simulink model "blob_analysis"  (Simulink 7.6)
settings: Solver=FixedStepDiscrete  StartTime=0.0  StopTime=0  FixedStep=1/30  RelTol=1e-3
values from neighbouring files (symbols this model uses):
  Iter_Segment_Thresh = 60    [VisionConstants.m]
undefined symbols (not defined in the file or in its folder): black_al, black_au, black_bl, black_bu, blue_al, blue_au, blue_bl, blue_bu, green_al, green_au, green_bl, green_bu, orange_al, orange_au, orange_bl, orange_bu, Rec, red_al, red_au, red_bl, red_bu, SDTV, white_al, white_au, white_bl, white_bu, yellow_al, yellow_au, yellow_bl, yellow_bu
libraries: vipgeotforms x21, vipconversions x14
(part 1 of 5)
settings Model: Creator=auvt  LastModifiedBy=auvt
settings RTWCC: TargetLang=C++

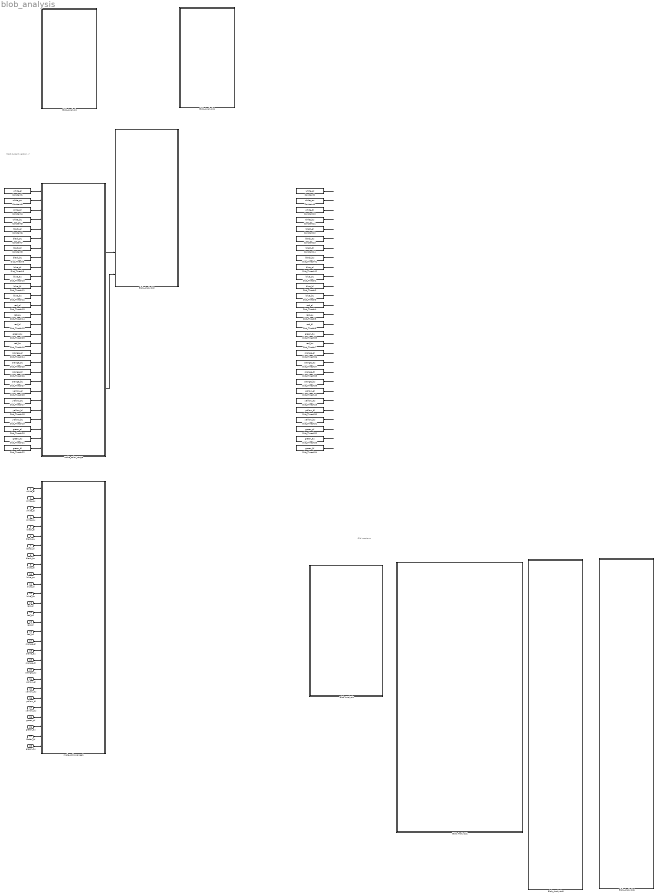
== system blob_analysis ==
  note: Old versions
  note: Most current version ->
  white_al : Inport
  white_au : Inport  Port=2
  white_bl : Inport  Port=3
  white_bu : Inport  Port=4
  black_al : Inport  Port=5
  black_au : Inport  Port=6
  black_bl : Inport  Port=7
  black_bu : Inport  Port=8
  blue_al : Inport  Port=9
  blue_au : Inport  Port=10
  blue_bl : Inport  Port=11
  blue_bu : Inport  Port=12
  red_al : Inport  Port=13
  red_au : Inport  Port=14
  red_bl : Inport  Port=15
  red_bu : Inport  Port=16
  orange_al : Inport  Port=17
  orane_au : Inport  Port=18
  orange_bl : Inport  Port=19
  orange_bu : Inport  Port=20
  yellow_al : Inport  Port=21
  yellow_au : Inport  Port=22
  yellow_bl : Inport  Port=23
  yellow_bu : Inport  Port=24
  green_al : Inport  Port=25
  green_au : Inport  Port=26
  breen_bl : Inport  Port=27
  green_bu : Inport  Port=28
  Blob Analysis : Subsystem
  Blob Analysis1 : Subsystem
  Blob_Analysis : Subsystem  TreatAsAtomicUnit=on
  Blob_Analysis1 : Subsystem  TreatAsAtomicUnit=on
  Blob_Analysis2 : Subsystem  TreatAsAtomicUnit=on
  Blob_Analysis5 : Subsystem  TreatAsAtomicUnit=on
  Blob_Analysis6 : Subsystem  TreatAsAtomicUnit=on
  Constant1 : Constant  Value=white_al  SampleTime=-1
  Constant10 : Constant  Value=white_bl  SampleTime=-1
  Constant11 : Constant  Value=white_bu  SampleTime=-1
  Constant12 : Constant  Value=black_al  SampleTime=-1
  Constant13 : Constant  Value=black_au  SampleTime=-1
  Constant14 : Constant  Value=black_bl  SampleTime=-1
  Constant2 : Constant  Value=white_al  SampleTime=-1
  Constant3 : Constant  Value=white_au  SampleTime=-1
  Constant4 : Constant  Value=white_bl  SampleTime=-1
  Constant5 : Constant  Value=white_bu  SampleTime=-1
  Constant6 : Constant  Value=black_al  SampleTime=-1
  Constant7 : Constant  Value=black_au  SampleTime=-1
  Constant8 : Constant  Value=black_bl  SampleTime=-1
  Constant9 : Constant  Value=white_au  SampleTime=-1
  Dist_Thresh1 : Constant  Value=blue_au  SampleTime=-1
  Dist_Thresh10 : Constant  Value=blue_au  SampleTime=-1
  Dist_Thresh11 : Constant  Value=blue_bl  SampleTime=-1
  Dist_Thresh12 : Constant  Value=blue_bu  SampleTime=-1
  Dist_Thresh13 : Constant  Value=red_al  SampleTime=-1
  Dist_Thresh14 : Constant  Value=red_au  SampleTime=-1
  Dist_Thresh15 : Constant  Value=red_bl  SampleTime=-1
  Dist_Thresh16 : Constant  Value=red_bu  SampleTime=-1
  Dist_Thresh17 : Constant  Value=yellow_au  SampleTime=-1
  Dist_Thresh18 : Constant  Value=yellow_bl  SampleTime=-1
  Dist_Thresh19 : Constant  Value=yellow_bu  SampleTime=-1
  Dist_Thresh2 : Constant  Value=blue_bl  SampleTime=-1
  Dist_Thresh20 : Constant  Value=green_al  SampleTime=-1
  Dist_Thresh21 : Constant  Value=green_au  SampleTime=-1
  Dist_Thresh22 : Constant  Value=green_bl  SampleTime=-1
  Dist_Thresh23 : Constant  Value=green_bu  SampleTime=-1
  Dist_Thresh24 : Constant  Value=orange_al  SampleTime=-1
  Dist_Thresh25 : Constant  Value=orange_au  SampleTime=-1
  Dist_Thresh26 : Constant  Value=orange_bl  SampleTime=-1
  Dist_Thresh27 : Constant  Value=orange_bu  SampleTime=-1
  Dist_Thresh28 : Constant  Value=yellow_al  SampleTime=-1
  Dist_Thresh29 : Constant  Value=yellow_au  SampleTime=-1
  Dist_Thresh3 : Constant  Value=blue_bu  SampleTime=-1
  Dist_Thresh30 : Constant  Value=yellow_bl  SampleTime=-1
  Dist_Thresh31 : Constant  Value=yellow_bu  SampleTime=-1
  Dist_Thresh32 : Constant  Value=green_al  SampleTime=-1
  Dist_Thresh33 : Constant  Value=green_au  SampleTime=-1
  Dist_Thresh34 : Constant  Value=green_bl  SampleTime=-1
  Dist_Thresh35 : Constant  Value=green_bu  SampleTime=-1
  Dist_Thresh36 : Constant  Value=orange_al  SampleTime=-1
  Dist_Thresh37 : Constant  Value=orange_au  SampleTime=-1
  Dist_Thresh38 : Constant  Value=orange_bl  SampleTime=-1
  Dist_Thresh39 : Constant  Value=orange_bu  SampleTime=-1
  Dist_Thresh4 : Constant  Value=red_al  SampleTime=-1
  Dist_Thresh40 : Constant  Value=yellow_al  SampleTime=-1
  Dist_Thresh41 : Constant  Value=black_bu  SampleTime=-1
  Dist_Thresh42 : Constant  Value=blue_al  SampleTime=-1
  Dist_Thresh5 : Constant  Value=red_au  SampleTime=-1
  Dist_Thresh6 : Constant  Value=red_bl  SampleTime=-1
  Dist_Thresh7 : Constant  Value=red_bu  SampleTime=-1
  Dist_Thresh8 : Constant  Value=black_bu  SampleTime=-1
  Dist_Thresh9 : Constant  Value=blue_al  SampleTime=-1
  make_color_range : Stateflow chart  TreatAsAtomicUnit=on
  make_color_range1 : Stateflow chart  TreatAsAtomicUnit=on
  wires:
  Constant1/1 -> make_color_range/1(white_al)
  Dist_Thresh22/1 -> make_color_range/28(green_bu)
  Constant3/1 -> make_color_range/2(white_au)
  Constant4/1 -> make_color_range/3(white_bl)
  Constant5/1 -> make_color_range/4(white_bu)
  Constant6/1 -> make_color_range/5(black_al)
  Constant7/1 -> make_color_range/6(black_au)
  Constant8/1 -> make_color_range/7(black_bl)
  Dist_Thresh8/1 -> make_color_range/8(black_bu)
  Dist_Thresh9/1 -> make_color_range/9(blue_al)
  Dist_Thresh10/1 -> make_color_range/10(blue_au)
  Dist_Thresh11/1 -> make_color_range/11(blue_bl)
  Dist_Thresh12/1 -> make_color_range/12(blue_bu)
  Dist_Thresh13/1 -> make_color_range/13(red_al)
  Dist_Thresh14/1 -> make_color_range/14(red_au)
  Dist_Thresh15/1 -> make_color_range/15(red_bl)
  Dist_Thresh23/1 -> make_color_range/16(red_bu)
  Dist_Thresh16/1 -> make_color_range/17(orange_al)
  Dist_Thresh24/1 -> make_color_range/18(orange_au)
  Dist_Thresh25/1 -> make_color_range/19(orange_bl)
  Dist_Thresh26/1 -> make_color_range/20(orange_bu)
  Dist_Thresh27/1 -> make_color_range/21(yellow_al)
  Dist_Thresh28/1 -> make_color_range/22(yellow_au)
  Dist_Thresh17/1 -> make_color_range/23(yellow_bl)
  Dist_Thresh18/1 -> make_color_range/24(yellow_bu)
  Dist_Thresh19/1 -> make_color_range/25(green_al)
  Dist_Thresh20/1 -> make_color_range/26(green_au)
  Dist_Thresh21/1 -> make_color_range/27(green_bl)
  Constant2/1 -> ?
  Dist_Thresh34/1 -> ?
  Constant9/1 -> ?
  Constant10/1 -> ?
  Constant11/1 -> ?
  Constant12/1 -> ?
  Constant13/1 -> ?
  Constant14/1 -> ?
  Dist_Thresh41/1 -> ?
  Dist_Thresh42/1 -> ?
  Dist_Thresh1/1 -> ?
  Dist_Thresh2/1 -> ?
  Dist_Thresh3/1 -> ?
  Dist_Thresh4/1 -> ?
  Dist_Thresh5/1 -> ?
  Dist_Thresh6/1 -> ?
  Dist_Thresh35/1 -> ?
  Dist_Thresh7/1 -> ?
  Dist_Thresh36/1 -> ?
  Dist_Thresh37/1 -> ?
  Dist_Thresh38/1 -> ?
  Dist_Thresh39/1 -> ?
  Dist_Thresh40/1 -> ?
  Dist_Thresh29/1 -> ?
  Dist_Thresh30/1 -> ?
  Dist_Thresh31/1 -> ?
  Dist_Thresh32/1 -> ?
  Dist_Thresh33/1 -> ?
  make_color_range/1(a_range) -> Blob_Analysis2/6(a_range)
  make_color_range/2(b_range) -> Blob_Analysis2/7(b_range)
  white_al/1 -> make_color_range1/1(white_al)
  white_au/1 -> make_color_range1/2(white_au)
  white_bl/1 -> make_color_range1/3(white_bl)
  white_bu/1 -> make_color_range1/4(white_bu)
  black_al/1 -> make_color_range1/5(black_al)
  black_au/1 -> make_color_range1/6(black_au)
  black_bl/1 -> make_color_range1/7(black_bl)
  black_bu/1 -> make_color_range1/8(black_bu)
  blue_al/1 -> make_color_range1/9(blue_al)
  blue_au/1 -> make_color_range1/10(blue_au)
  blue_bl/1 -> make_color_range1/11(blue_bl)
  blue_bu/1 -> make_color_range1/12(blue_bu)
  red_al/1 -> make_color_range1/13(red_al)
  red_au/1 -> make_color_range1/14(red_au)
  red_bl/1 -> make_color_range1/15(red_bl)
  red_bu/1 -> make_color_range1/16(red_bu)
  orange_al/1 -> make_color_range1/17(orange_al)
  orane_au/1 -> make_color_range1/18(orange_au)
  orange_bl/1 -> make_color_range1/19(orange_bl)
  orange_bu/1 -> make_color_range1/20(orange_bu)
  yellow_al/1 -> make_color_range1/21(yellow_al)
  yellow_au/1 -> make_color_range1/22(yellow_au)
  yellow_bl/1 -> make_color_range1/23(yellow_bl)
  yellow_bu/1 -> make_color_range1/24(yellow_bu)
  green_al/1 -> make_color_range1/25(green_al)
  green_au/1 -> make_color_range1/26(green_au)
  breen_bl/1 -> make_color_range1/27(green_bl)
  green_bu/1 -> make_color_range1/28(green_bu)

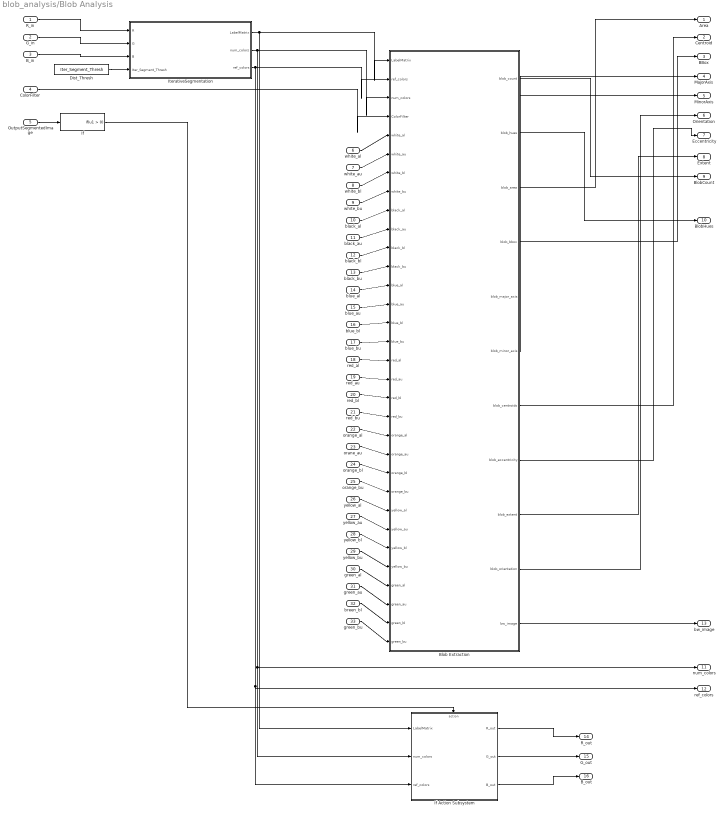
== system blob_analysis/Blob Analysis ==
  R_in : Inport
  G_in : Inport  Port=2
  B_in : Inport  Port=3
  ColorFilter : Inport  Port=4
  OutputSegmentedImage : Inport  Port=5
  white_al : Inport  Port=6
  white_au : Inport  Port=7
  white_bl : Inport  Port=8
  white_bu : Inport  Port=9
  black_al : Inport  Port=10
  black_au : Inport  Port=11
  black_bl : Inport  Port=12
  black_bu : Inport  Port=13
  blue_al : Inport  Port=14
  blue_au : Inport  Port=15
  blue_bl : Inport  Port=16
  blue_bu : Inport  Port=17
  red_al : Inport  Port=18
  red_au : Inport  Port=19
  red_bl : Inport  Port=20
  red_bu : Inport  Port=21
  orange_al : Inport  Port=22
  orane_au : Inport  Port=23
  orange_bl : Inport  Port=24
  orange_bu : Inport  Port=25
  yellow_al : Inport  Port=26
  yellow_au : Inport  Port=27
  yellow_bl : Inport  Port=28
  yellow_bu : Inport  Port=29
  green_al : Inport  Port=30
  green_au : Inport  Port=31
  breen_bl : Inport  Port=32
  green_bu : Inport  Port=33
  Blob Extraction : Stateflow chart  TreatAsAtomicUnit=on
  Dist_Thresh : Constant  Value=Iter_Segment_Thresh  SampleTime=-1
  If : If  ShowElse=off
  If Action Subsystem : Subsystem  TreatAsAtomicUnit=on
  IterativeSegmentation : Subsystem
      settings: UndoDeleteFcn=Stateflow.SLINSF.SimulinkMan.restorePreDeleteFcn  PreDeleteFcn=Stateflow.SLINSF.SimulinkMan.removePreDeleteFcn
  Area : Outport
  Centroid : Outport  Port=2
  BBox : Outport  Port=3
  MajorAxis : Outport  Port=4
  MinorAxis : Outport  Port=5
  Orientation : Outport  Port=6
  Eccentricity : Outport  Port=7
  Extent : Outport  Port=8
  BlobCount : Outport  Port=9
  BlobHues : Outport  Port=10
  num_colors : Outport  Port=11
  ref_colors : Outport  Port=12
  bw_image : Outport  Port=13
  R_out : Outport  Port=14
  G_out : Outport  Port=15
  B_out : Outport  Port=16
  wires:
  IterativeSegmentation/1(LabelMatrix) -> Blob Extraction/1(LabelMatrix), If Action Subsystem/1(LabelMatrix)
  IterativeSegmentation/2(num_colors) -> Blob Extraction/3(num_colors), If Action Subsystem/2(num_colors), num_colors/1
  IterativeSegmentation/3(ref_colors) -> Blob Extraction/2(ref_colors), If Action Subsystem/3(ref_colors), ref_colors/1
  Blob Extraction/3(blob_area) -> Area/1
  Blob Extraction/7(blob_centroids) -> Centroid/1
  Blob Extraction/4(blob_bbox) -> BBox/1
  Blob Extraction/5(blob_major_axis) -> MajorAxis/1
  Blob Extraction/6(blob_minor_axis) -> MinorAxis/1
  Blob Extraction/10(blob_orientation) -> Orientation/1
  Blob Extraction/8(blob_eccentricity) -> Eccentricity/1
  Blob Extraction/9(blob_extent) -> Extent/1
  Blob Extraction/1(blob_count) -> BlobCount/1
  Blob Extraction/2(blob_hues) -> BlobHues/1
  ColorFilter/1 -> Blob Extraction/4(ColorFilter)
  Dist_Thresh/1 -> IterativeSegmentation/4(Iter_Segment_Thresh)
  R_in/1 -> IterativeSegmentation/1(R)
  G_in/1 -> IterativeSegmentation/2(G)
  B_in/1 -> IterativeSegmentation/3(B)
  white_al/1 -> Blob Extraction/5(white_al)
  white_au/1 -> Blob Extraction/6(white_au)
  white_bl/1 -> Blob Extraction/7(white_bl)
  white_bu/1 -> Blob Extraction/8(white_bu)
  black_al/1 -> Blob Extraction/9(black_al)
  black_au/1 -> Blob Extraction/10(black_au)
  black_bl/1 -> Blob Extraction/11(black_bl)
  black_bu/1 -> Blob Extraction/12(black_bu)
  blue_al/1 -> Blob Extraction/13(blue_al)
  blue_au/1 -> Blob Extraction/14(blue_au)
  blue_bl/1 -> Blob Extraction/15(blue_bl)
  blue_bu/1 -> Blob Extraction/16(blue_bu)
  red_al/1 -> Blob Extraction/17(red_al)
  red_au/1 -> Blob Extraction/18(red_au)
  red_bl/1 -> Blob Extraction/19(red_bl)
  red_bu/1 -> Blob Extraction/20(red_bu)
  orange_al/1 -> Blob Extraction/21(orange_al)
  orane_au/1 -> Blob Extraction/22(orange_au)
  orange_bl/1 -> Blob Extraction/23(orange_bl)
  orange_bu/1 -> Blob Extraction/24(orange_bu)
  yellow_al/1 -> Blob Extraction/25(yellow_al)
  yellow_au/1 -> Blob Extraction/26(yellow_au)
  yellow_bl/1 -> Blob Extraction/27(yellow_bl)
  yellow_bu/1 -> Blob Extraction/28(yellow_bu)
  green_al/1 -> Blob Extraction/29(green_al)
  green_au/1 -> Blob Extraction/30(green_au)
  breen_bl/1 -> Blob Extraction/31(green_bl)
  green_bu/1 -> Blob Extraction/32(green_bu)
  If/1 -> If Action Subsystem/Action
  OutputSegmentedImage/1 -> If/1
  If Action Subsystem/1(R_out) -> R_out/1
  If Action Subsystem/2(G_out) -> G_out/1
  If Action Subsystem/3(B_out) -> B_out/1
  Blob Extraction/11(bw_image) -> bw_image/1

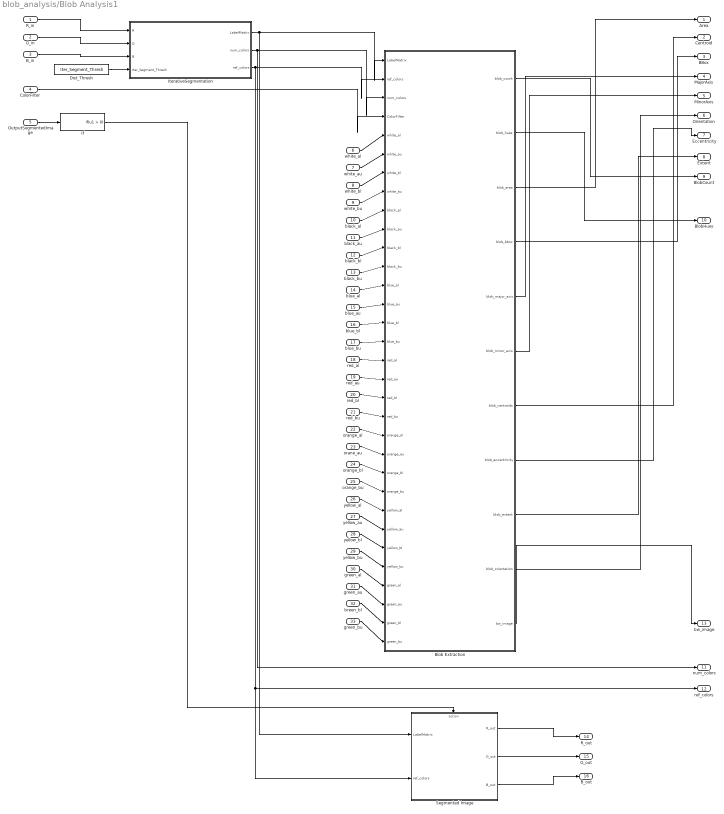
== system blob_analysis/Blob Analysis1 ==
  R_in : Inport
  G_in : Inport  Port=2
  B_in : Inport  Port=3
  ColorFilter : Inport  Port=4
  OutputSegmentedImage : Inport  Port=5
  white_al : Inport  Port=6
  white_au : Inport  Port=7
  white_bl : Inport  Port=8
  white_bu : Inport  Port=9
  black_al : Inport  Port=10
  black_au : Inport  Port=11
  black_bl : Inport  Port=12
  black_bu : Inport  Port=13
  blue_al : Inport  Port=14
  blue_au : Inport  Port=15
  blue_bl : Inport  Port=16
  blue_bu : Inport  Port=17
  red_al : Inport  Port=18
  red_au : Inport  Port=19
  red_bl : Inport  Port=20
  red_bu : Inport  Port=21
  orange_al : Inport  Port=22
  orane_au : Inport  Port=23
  orange_bl : Inport  Port=24
  orange_bu : Inport  Port=25
  yellow_al : Inport  Port=26
  yellow_au : Inport  Port=27
  yellow_bl : Inport  Port=28
  yellow_bu : Inport  Port=29
  green_al : Inport  Port=30
  green_au : Inport  Port=31
  breen_bl : Inport  Port=32
  green_bu : Inport  Port=33
  Blob Extraction : Stateflow chart  TreatAsAtomicUnit=on
  Dist_Thresh : Constant  Value=Iter_Segment_Thresh  SampleTime=-1
  If : If  ShowElse=off
  IterativeSegmentation : Subsystem
      settings: UndoDeleteFcn=Stateflow.SLINSF.SimulinkMan.restorePreDeleteFcn  PreDeleteFcn=Stateflow.SLINSF.SimulinkMan.removePreDeleteFcn
  Segmented Image : Subsystem  TreatAsAtomicUnit=on
  Area : Outport
  Centroid : Outport  Port=2
  BBox : Outport  Port=3
  MajorAxis : Outport  Port=4
  MinorAxis : Outport  Port=5
  Orientation : Outport  Port=6
  Eccentricity : Outport  Port=7
  Extent : Outport  Port=8
  BlobCount : Outport  Port=9
  BlobHues : Outport  Port=10
  num_colors : Outport  Port=11
  ref_colors : Outport  Port=12
  bw_image : Outport  Port=13
  R_out : Outport  Port=14
  G_out : Outport  Port=15
  B_out : Outport  Port=16
  wires:
  IterativeSegmentation/1(LabelMatrix) -> Blob Extraction/1(LabelMatrix), Segmented Image/1(LabelMatrix)
  IterativeSegmentation/2(num_colors) -> Blob Extraction/3(num_colors), num_colors/1
  IterativeSegmentation/3(ref_colors) -> Blob Extraction/2(ref_colors), Segmented Image/2(ref_colors), ref_colors/1
  Blob Extraction/3(blob_area) -> Area/1
  Blob Extraction/7(blob_centroids) -> Centroid/1
  Blob Extraction/4(blob_bbox) -> BBox/1
  Blob Extraction/5(blob_major_axis) -> MajorAxis/1
  Blob Extraction/6(blob_minor_axis) -> MinorAxis/1
  Blob Extraction/10(blob_orientation) -> Orientation/1
  Blob Extraction/8(blob_eccentricity) -> Eccentricity/1
  Blob Extraction/9(blob_extent) -> Extent/1
  Blob Extraction/1(blob_count) -> BlobCount/1
  Blob Extraction/2(blob_hues) -> BlobHues/1
  ColorFilter/1 -> Blob Extraction/4(ColorFilter)
  Dist_Thresh/1 -> IterativeSegmentation/4(Iter_Segment_Thresh)
  R_in/1 -> IterativeSegmentation/1(R)
  G_in/1 -> IterativeSegmentation/2(G)
  B_in/1 -> IterativeSegmentation/3(B)
  white_al/1 -> Blob Extraction/5(white_al)
  white_au/1 -> Blob Extraction/6(white_au)
  white_bl/1 -> Blob Extraction/7(white_bl)
  white_bu/1 -> Blob Extraction/8(white_bu)
  black_al/1 -> Blob Extraction/9(black_al)
  black_au/1 -> Blob Extraction/10(black_au)
  black_bl/1 -> Blob Extraction/11(black_bl)
  black_bu/1 -> Blob Extraction/12(black_bu)
  blue_al/1 -> Blob Extraction/13(blue_al)
  blue_au/1 -> Blob Extraction/14(blue_au)
  blue_bl/1 -> Blob Extraction/15(blue_bl)
  blue_bu/1 -> Blob Extraction/16(blue_bu)
  red_al/1 -> Blob Extraction/17(red_al)
  red_au/1 -> Blob Extraction/18(red_au)
  red_bl/1 -> Blob Extraction/19(red_bl)
  red_bu/1 -> Blob Extraction/20(red_bu)
  orange_al/1 -> Blob Extraction/21(orange_al)
  orane_au/1 -> Blob Extraction/22(orange_au)
  orange_bl/1 -> Blob Extraction/23(orange_bl)
  orange_bu/1 -> Blob Extraction/24(orange_bu)
  yellow_al/1 -> Blob Extraction/25(yellow_al)
  yellow_au/1 -> Blob Extraction/26(yellow_au)
  yellow_bl/1 -> Blob Extraction/27(yellow_bl)
  yellow_bu/1 -> Blob Extraction/28(yellow_bu)
  green_al/1 -> Blob Extraction/29(green_al)
  green_au/1 -> Blob Extraction/30(green_au)
  breen_bl/1 -> Blob Extraction/31(green_bl)
  green_bu/1 -> Blob Extraction/32(green_bu)
  If/1 -> Segmented Image/Action
  OutputSegmentedImage/1 -> If/1
  Segmented Image/1(R_out) -> R_out/1
  Segmented Image/2(G_out) -> G_out/1
  Segmented Image/3(B_out) -> B_out/1
  Blob Extraction/11(bw_image) -> bw_image/1

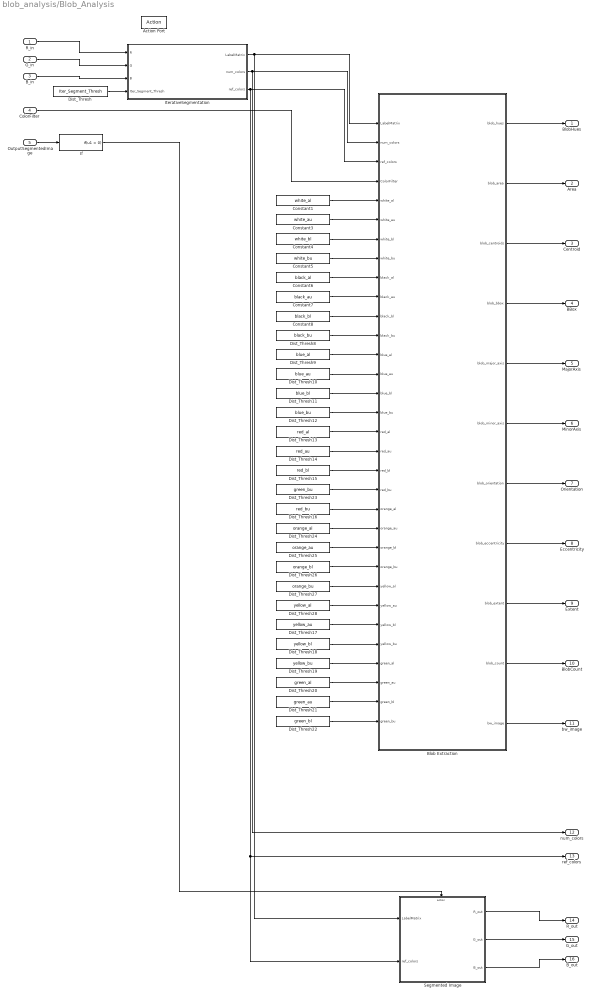
== system blob_analysis/Blob_Analysis ==
  R_in : Inport
  G_in : Inport  Port=2
  B_in : Inport  Port=3
  ColorFilter : Inport  Port=4
  OutputSegmentedImage : Inport  Port=5
  Action Port : ActionPort
  Blob Extraction : Stateflow chart  TreatAsAtomicUnit=on
  Constant1 : Constant  Value=white_al  SampleTime=-1
  Constant3 : Constant  Value=white_au  SampleTime=-1
  Constant4 : Constant  Value=white_bl  SampleTime=-1
  Constant5 : Constant  Value=white_bu  SampleTime=-1
  Constant6 : Constant  Value=black_al  SampleTime=-1
  Constant7 : Constant  Value=black_au  SampleTime=-1
  Constant8 : Constant  Value=black_bl  SampleTime=-1
  Dist_Thresh : Constant  Value=Iter_Segment_Thresh  SampleTime=-1
  Dist_Thresh10 : Constant  Value=blue_au  SampleTime=-1
  Dist_Thresh11 : Constant  Value=blue_bl  SampleTime=-1
  Dist_Thresh12 : Constant  Value=blue_bu  SampleTime=-1
  Dist_Thresh13 : Constant  Value=red_al  SampleTime=-1
  Dist_Thresh14 : Constant  Value=red_au  SampleTime=-1
  Dist_Thresh15 : Constant  Value=red_bl  SampleTime=-1
  Dist_Thresh16 : Constant  Value=red_bu  SampleTime=-1
  Dist_Thresh17 : Constant  Value=yellow_au  SampleTime=-1
  Dist_Thresh18 : Constant  Value=yellow_bl  SampleTime=-1
  Dist_Thresh19 : Constant  Value=yellow_bu  SampleTime=-1
  Dist_Thresh20 : Constant  Value=green_al  SampleTime=-1
  Dist_Thresh21 : Constant  Value=green_au  SampleTime=-1
  Dist_Thresh22 : Constant  Value=green_bl  SampleTime=-1
  Dist_Thresh23 : Constant  Value=green_bu  SampleTime=-1
  Dist_Thresh24 : Constant  Value=orange_al  SampleTime=-1
  Dist_Thresh25 : Constant  Value=orange_au  SampleTime=-1
  Dist_Thresh26 : Constant  Value=orange_bl  SampleTime=-1
  Dist_Thresh27 : Constant  Value=orange_bu  SampleTime=-1
  Dist_Thresh28 : Constant  Value=yellow_al  SampleTime=-1
  Dist_Thresh8 : Constant  Value=black_bu  SampleTime=-1
  Dist_Thresh9 : Constant  Value=blue_al  SampleTime=-1
  If : If  ShowElse=off
  IterativeSegmentation : Subsystem
      settings: UndoDeleteFcn=Stateflow.SLINSF.SimulinkMan.restorePreDeleteFcn  PreDeleteFcn=Stateflow.SLINSF.SimulinkMan.removePreDeleteFcn
  Segmented Image : Subsystem  TreatAsAtomicUnit=on
  BlobHues : Outport
  Area : Outport  Port=2
  Centroid : Outport  Port=3
  BBox : Outport  Port=4
  MajorAxis : Outport  Port=5
  MinorAxis : Outport  Port=6
  Orientation : Outport  Port=7
  Eccentricity : Outport  Port=8
  Extent : Outport  Port=9
  BlobCount : Outport  Port=10
  bw_image : Outport  Port=11
  num_colors : Outport  Port=12
  ref_colors : Outport  Port=13
  R_out : Outport  Port=14
  G_out : Outport  Port=15
  B_out : Outport  Port=16
  wires:
  Segmented Image/3(B_out) -> B_out/1
  Segmented Image/2(G_out) -> G_out/1
  Segmented Image/1(R_out) -> R_out/1
  OutputSegmentedImage/1 -> If/1
  If/1 -> Segmented Image/Action
  B_in/1 -> IterativeSegmentation/3(B)
  G_in/1 -> IterativeSegmentation/2(G)
  R_in/1 -> IterativeSegmentation/1(R)
  Dist_Thresh/1 -> IterativeSegmentation/4(Iter_Segment_Thresh)
  IterativeSegmentation/3(ref_colors) -> ref_colors/1, Segmented Image/2(ref_colors), Blob Extraction/3(ref_colors)
  IterativeSegmentation/2(num_colors) -> num_colors/1, Blob Extraction/2(num_colors)
  IterativeSegmentation/1(LabelMatrix) -> Segmented Image/1(LabelMatrix), Blob Extraction/1(LabelMatrix)
  Dist_Thresh22/1 -> Blob Extraction/32(green_bu)
  Dist_Thresh21/1 -> Blob Extraction/31(green_bl)
  Dist_Thresh20/1 -> Blob Extraction/30(green_au)
  Dist_Thresh19/1 -> Blob Extraction/29(green_al)
  Dist_Thresh18/1 -> Blob Extraction/28(yellow_bu)
  Dist_Thresh17/1 -> Blob Extraction/27(yellow_bl)
  Dist_Thresh28/1 -> Blob Extraction/26(yellow_au)
  Dist_Thresh27/1 -> Blob Extraction/25(yellow_al)
  Dist_Thresh26/1 -> Blob Extraction/24(orange_bu)
  Dist_Thresh25/1 -> Blob Extraction/23(orange_bl)
  Dist_Thresh24/1 -> Blob Extraction/22(orange_au)
  Dist_Thresh16/1 -> Blob Extraction/21(orange_al)
  Dist_Thresh23/1 -> Blob Extraction/20(red_bu)
  Dist_Thresh15/1 -> Blob Extraction/19(red_bl)
  Dist_Thresh14/1 -> Blob Extraction/18(red_au)
  Dist_Thresh13/1 -> Blob Extraction/17(red_al)
  Dist_Thresh12/1 -> Blob Extraction/16(blue_bu)
  Dist_Thresh11/1 -> Blob Extraction/15(blue_bl)
  Dist_Thresh10/1 -> Blob Extraction/14(blue_au)
  Dist_Thresh9/1 -> Blob Extraction/13(blue_al)
  Dist_Thresh8/1 -> Blob Extraction/12(black_bu)
  Constant8/1 -> Blob Extraction/11(black_bl)
  Constant7/1 -> Blob Extraction/10(black_au)
  Constant6/1 -> Blob Extraction/9(black_al)
  Constant5/1 -> Blob Extraction/8(white_bu)
  Constant4/1 -> Blob Extraction/7(white_bl)
  Constant3/1 -> Blob Extraction/6(white_au)
  Constant1/1 -> Blob Extraction/5(white_al)
  ColorFilter/1 -> Blob Extraction/4(ColorFilter)
  Blob Extraction/1(blob_hues) -> BlobHues/1
  Blob Extraction/2(blob_area) -> Area/1
  Blob Extraction/3(blob_centroids) -> Centroid/1
  Blob Extraction/4(blob_bbox) -> BBox/1
  Blob Extraction/5(blob_major_axis) -> MajorAxis/1
  Blob Extraction/6(blob_minor_axis) -> MinorAxis/1
  Blob Extraction/7(blob_orientation) -> Orientation/1
  Blob Extraction/8(blob_eccentricity) -> Eccentricity/1
  Blob Extraction/9(blob_extent) -> Extent/1
  Blob Extraction/10(blob_count) -> BlobCount/1
  Blob Extraction/11(bw_image) -> bw_image/1

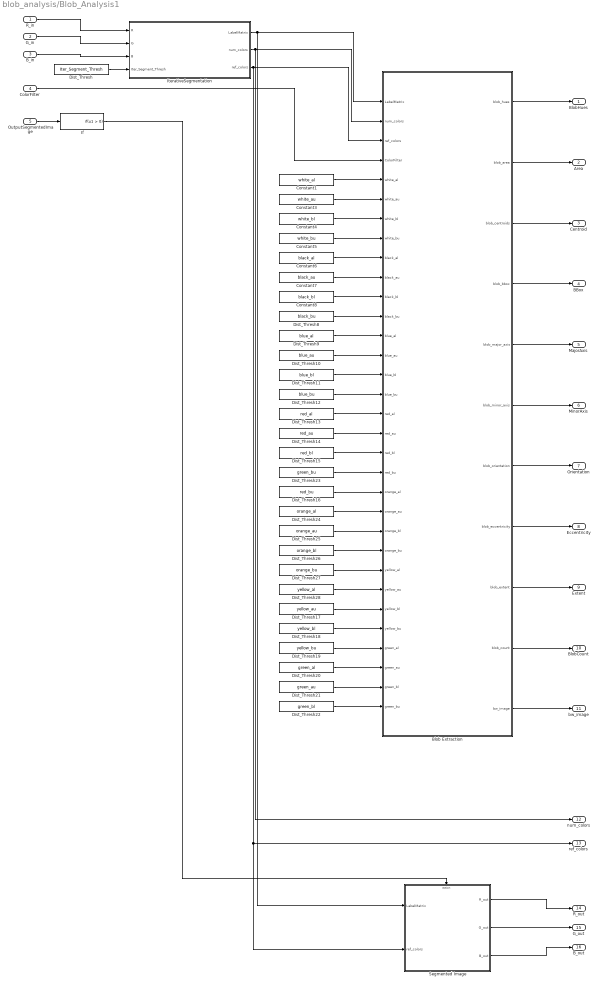
== system blob_analysis/Blob_Analysis1 ==
  R_in : Inport
  G_in : Inport  Port=2
  B_in : Inport  Port=3
  ColorFilter : Inport  Port=4
  OutputSegmentedImage : Inport  Port=5
  Blob Extraction : Stateflow chart  TreatAsAtomicUnit=on
  Constant1 : Constant  Value=white_al  SampleTime=-1
  Constant3 : Constant  Value=white_au  SampleTime=-1
  Constant4 : Constant  Value=white_bl  SampleTime=-1
  Constant5 : Constant  Value=white_bu  SampleTime=-1
  Constant6 : Constant  Value=black_al  SampleTime=-1
  Constant7 : Constant  Value=black_au  SampleTime=-1
  Constant8 : Constant  Value=black_bl  SampleTime=-1
  Dist_Thresh : Constant  Value=Iter_Segment_Thresh  SampleTime=-1
  Dist_Thresh10 : Constant  Value=blue_au  SampleTime=-1
  Dist_Thresh11 : Constant  Value=blue_bl  SampleTime=-1
  Dist_Thresh12 : Constant  Value=blue_bu  SampleTime=-1
  Dist_Thresh13 : Constant  Value=red_al  SampleTime=-1
  Dist_Thresh14 : Constant  Value=red_au  SampleTime=-1
  Dist_Thresh15 : Constant  Value=red_bl  SampleTime=-1
  Dist_Thresh16 : Constant  Value=red_bu  SampleTime=-1
  Dist_Thresh17 : Constant  Value=yellow_au  SampleTime=-1
  Dist_Thresh18 : Constant  Value=yellow_bl  SampleTime=-1
  Dist_Thresh19 : Constant  Value=yellow_bu  SampleTime=-1
  Dist_Thresh20 : Constant  Value=green_al  SampleTime=-1
  Dist_Thresh21 : Constant  Value=green_au  SampleTime=-1
  Dist_Thresh22 : Constant  Value=green_bl  SampleTime=-1
  Dist_Thresh23 : Constant  Value=green_bu  SampleTime=-1
  Dist_Thresh24 : Constant  Value=orange_al  SampleTime=-1
  Dist_Thresh25 : Constant  Value=orange_au  SampleTime=-1
  Dist_Thresh26 : Constant  Value=orange_bl  SampleTime=-1
  Dist_Thresh27 : Constant  Value=orange_bu  SampleTime=-1
  Dist_Thresh28 : Constant  Value=yellow_al  SampleTime=-1
  Dist_Thresh8 : Constant  Value=black_bu  SampleTime=-1
  Dist_Thresh9 : Constant  Value=blue_al  SampleTime=-1
  If : If  ShowElse=off
  IterativeSegmentation : Subsystem
      settings: UndoDeleteFcn=Stateflow.SLINSF.SimulinkMan.restorePreDeleteFcn  PreDeleteFcn=Stateflow.SLINSF.SimulinkMan.removePreDeleteFcn
  Segmented Image : Subsystem  TreatAsAtomicUnit=on
  BlobHues : Outport
  Area : Outport  Port=2
  Centroid : Outport  Port=3
  BBox : Outport  Port=4
  MajorAxis : Outport  Port=5
  MinorAxis : Outport  Port=6
  Orientation : Outport  Port=7
  Eccentricity : Outport  Port=8
  Extent : Outport  Port=9
  BlobCount : Outport  Port=10
  bw_image : Outport  Port=11
  num_colors : Outport  Port=12
  ref_colors : Outport  Port=13
  R_out : Outport  Port=14
  G_out : Outport  Port=15
  B_out : Outport  Port=16
  wires:
  Blob Extraction/11(bw_image) -> bw_image/1
  Blob Extraction/10(blob_count) -> BlobCount/1
  Blob Extraction/9(blob_extent) -> Extent/1
  Blob Extraction/8(blob_eccentricity) -> Eccentricity/1
  Blob Extraction/7(blob_orientation) -> Orientation/1
  Blob Extraction/6(blob_minor_axis) -> MinorAxis/1
  Blob Extraction/5(blob_major_axis) -> MajorAxis/1
  Blob Extraction/4(blob_bbox) -> BBox/1
  Blob Extraction/3(blob_centroids) -> Centroid/1
  Blob Extraction/2(blob_area) -> Area/1
  Blob Extraction/1(blob_hues) -> BlobHues/1
  ColorFilter/1 -> Blob Extraction/4(ColorFilter)
  Constant1/1 -> Blob Extraction/5(white_al)
  Constant3/1 -> Blob Extraction/6(white_au)
  Constant4/1 -> Blob Extraction/7(white_bl)
  Constant5/1 -> Blob Extraction/8(white_bu)
  Constant6/1 -> Blob Extraction/9(black_al)
  Constant7/1 -> Blob Extraction/10(black_au)
  Constant8/1 -> Blob Extraction/11(black_bl)
  Dist_Thresh8/1 -> Blob Extraction/12(black_bu)
  Dist_Thresh9/1 -> Blob Extraction/13(blue_al)
  Dist_Thresh10/1 -> Blob Extraction/14(blue_au)
  Dist_Thresh11/1 -> Blob Extraction/15(blue_bl)
  Dist_Thresh12/1 -> Blob Extraction/16(blue_bu)
  Dist_Thresh13/1 -> Blob Extraction/17(red_al)
  Dist_Thresh14/1 -> Blob Extraction/18(red_au)
  Dist_Thresh15/1 -> Blob Extraction/19(red_bl)
  Dist_Thresh23/1 -> Blob Extraction/20(red_bu)
  Dist_Thresh16/1 -> Blob Extraction/21(orange_al)
  Dist_Thresh24/1 -> Blob Extraction/22(orange_au)
  Dist_Thresh25/1 -> Blob Extraction/23(orange_bl)
  Dist_Thresh26/1 -> Blob Extraction/24(orange_bu)
  Dist_Thresh27/1 -> Blob Extraction/25(yellow_al)
  Dist_Thresh28/1 -> Blob Extraction/26(yellow_au)
  Dist_Thresh17/1 -> Blob Extraction/27(yellow_bl)
  Dist_Thresh18/1 -> Blob Extraction/28(yellow_bu)
  Dist_Thresh19/1 -> Blob Extraction/29(green_al)
  Dist_Thresh20/1 -> Blob Extraction/30(green_au)
  Dist_Thresh21/1 -> Blob Extraction/31(green_bl)
  Dist_Thresh22/1 -> Blob Extraction/32(green_bu)
  IterativeSegmentation/1(LabelMatrix) -> Blob Extraction/1(LabelMatrix), Segmented Image/1(LabelMatrix)
  IterativeSegmentation/2(num_colors) -> Blob Extraction/2(num_colors), num_colors/1
  IterativeSegmentation/3(ref_colors) -> Blob Extraction/3(ref_colors), Segmented Image/2(ref_colors), ref_colors/1
  Dist_Thresh/1 -> IterativeSegmentation/4(Iter_Segment_Thresh)
  R_in/1 -> IterativeSegmentation/1(R)
  G_in/1 -> IterativeSegmentation/2(G)
  B_in/1 -> IterativeSegmentation/3(B)
  If/1 -> Segmented Image/Action
  OutputSegmentedImage/1 -> If/1
  Segmented Image/1(R_out) -> R_out/1
  Segmented Image/2(G_out) -> G_out/1
  Segmented Image/3(B_out) -> B_out/1

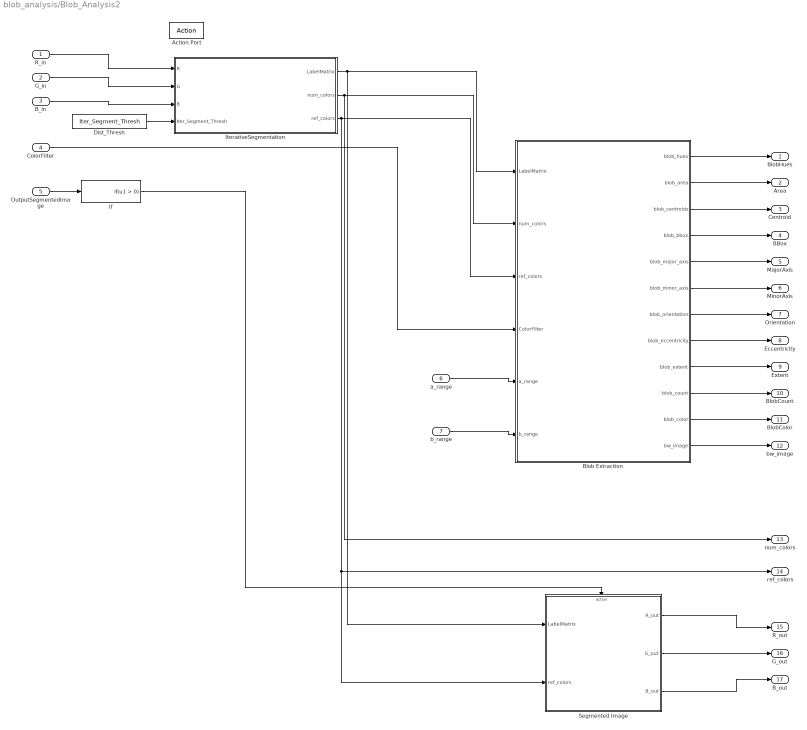
== system blob_analysis/Blob_Analysis2 ==
  R_in : Inport
  G_in : Inport  Port=2
  B_in : Inport  Port=3
  ColorFilter : Inport  Port=4
  OutputSegmentedImage : Inport  Port=5
  a_range : Inport  Port=6
  b_range : Inport  Port=7
  Action Port : ActionPort
  Blob Extraction : Stateflow chart  TreatAsAtomicUnit=on
  Dist_Thresh : Constant  Value=Iter_Segment_Thresh  SampleTime=-1
  If : If  ShowElse=off
  IterativeSegmentation : Subsystem
      settings: UndoDeleteFcn=Stateflow.SLINSF.SimulinkMan.restorePreDeleteFcn  PreDeleteFcn=Stateflow.SLINSF.SimulinkMan.removePreDeleteFcn
  Segmented Image : Subsystem  TreatAsAtomicUnit=on
  BlobHues : Outport
  Area : Outport  Port=2
  Centroid : Outport  Port=3
  BBox : Outport  Port=4
  MajorAxis : Outport  Port=5
  MinorAxis : Outport  Port=6
  Orientation : Outport  Port=7
  Eccentricity : Outport  Port=8
  Extent : Outport  Port=9
  BlobCount : Outport  Port=10
  BlobColor : Outport  Port=11
  bw_image : Outport  Port=12
  num_colors : Outport  Port=13
  ref_colors : Outport  Port=14
  R_out : Outport  Port=15
  G_out : Outport  Port=16
  B_out : Outport  Port=17
  wires:
  Blob Extraction/12(bw_image) -> bw_image/1
  Blob Extraction/10(blob_count) -> BlobCount/1
  Blob Extraction/9(blob_extent) -> Extent/1
  Blob Extraction/8(blob_eccentricity) -> Eccentricity/1
  Blob Extraction/7(blob_orientation) -> Orientation/1
  Blob Extraction/6(blob_minor_axis) -> MinorAxis/1
  Blob Extraction/5(blob_major_axis) -> MajorAxis/1
  Blob Extraction/4(blob_bbox) -> BBox/1
  Blob Extraction/3(blob_centroids) -> Centroid/1
  Blob Extraction/2(blob_area) -> Area/1
  Blob Extraction/1(blob_hues) -> BlobHues/1
  ColorFilter/1 -> Blob Extraction/4(ColorFilter)
  a_range/1 -> Blob Extraction/5(a_range)
  b_range/1 -> Blob Extraction/6(b_range)
  IterativeSegmentation/1(LabelMatrix) -> Blob Extraction/1(LabelMatrix), Segmented Image/1(LabelMatrix)
  IterativeSegmentation/2(num_colors) -> Blob Extraction/2(num_colors), num_colors/1
  IterativeSegmentation/3(ref_colors) -> Blob Extraction/3(ref_colors), Segmented Image/2(ref_colors), ref_colors/1
  Dist_Thresh/1 -> IterativeSegmentation/4(Iter_Segment_Thresh)
  R_in/1 -> IterativeSegmentation/1(R)
  G_in/1 -> IterativeSegmentation/2(G)
  B_in/1 -> IterativeSegmentation/3(B)
  If/1 -> Segmented Image/Action
  OutputSegmentedImage/1 -> If/1
  Segmented Image/1(R_out) -> R_out/1
  Segmented Image/2(G_out) -> G_out/1
  Segmented Image/3(B_out) -> B_out/1
  Blob Extraction/11(blob_color) -> BlobColor/1

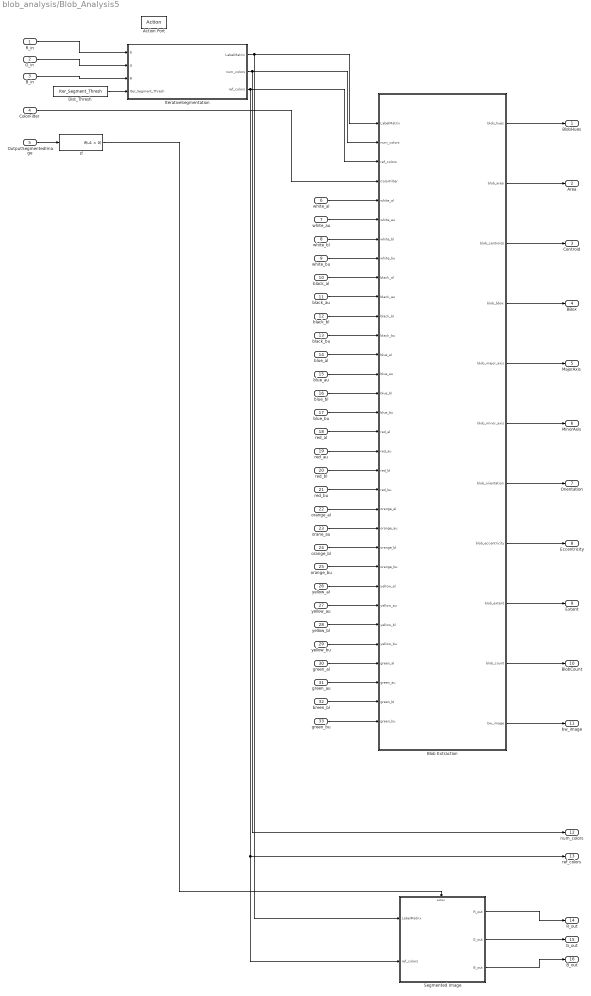
== system blob_analysis/Blob_Analysis5 ==
  R_in : Inport
  G_in : Inport  Port=2
  B_in : Inport  Port=3
  ColorFilter : Inport  Port=4
  OutputSegmentedImage : Inport  Port=5
  white_al : Inport  Port=6
  white_au : Inport  Port=7
  white_bl : Inport  Port=8
  white_bu : Inport  Port=9
  black_al : Inport  Port=10
  black_au : Inport  Port=11
  black_bl : Inport  Port=12
  black_bu : Inport  Port=13
  blue_al : Inport  Port=14
  blue_au : Inport  Port=15
  blue_bl : Inport  Port=16
  blue_bu : Inport  Port=17
  red_al : Inport  Port=18
  red_au : Inport  Port=19
  red_bl : Inport  Port=20
  red_bu : Inport  Port=21
  orange_al : Inport  Port=22
  orane_au : Inport  Port=23
  orange_bl : Inport  Port=24
  orange_bu : Inport  Port=25
  yellow_al : Inport  Port=26
  yellow_au : Inport  Port=27
  yellow_bl : Inport  Port=28
  yellow_bu : Inport  Port=29
  green_al : Inport  Port=30
  green_au : Inport  Port=31
  breen_bl : Inport  Port=32
  green_bu : Inport  Port=33
  Action Port : ActionPort
  Blob Extraction : Stateflow chart  TreatAsAtomicUnit=on
  Dist_Thresh : Constant  Value=Iter_Segment_Thresh  SampleTime=-1
  If : If  ShowElse=off
  IterativeSegmentation : Subsystem
      settings: UndoDeleteFcn=Stateflow.SLINSF.SimulinkMan.restorePreDeleteFcn  PreDeleteFcn=Stateflow.SLINSF.SimulinkMan.removePreDeleteFcn
  Segmented Image : Subsystem  TreatAsAtomicUnit=on
  BlobHues : Outport
  Area : Outport  Port=2
  Centroid : Outport  Port=3
  BBox : Outport  Port=4
  MajorAxis : Outport  Port=5
  MinorAxis : Outport  Port=6
  Orientation : Outport  Port=7
  Eccentricity : Outport  Port=8
  Extent : Outport  Port=9
  BlobCount : Outport  Port=10
  bw_image : Outport  Port=11
  num_colors : Outport  Port=12
  ref_colors : Outport  Port=13
  R_out : Outport  Port=14
  G_out : Outport  Port=15
  B_out : Outport  Port=16
  wires:
  Blob Extraction/11(bw_image) -> bw_image/1
  Blob Extraction/10(blob_count) -> BlobCount/1
  Blob Extraction/9(blob_extent) -> Extent/1
  Blob Extraction/8(blob_eccentricity) -> Eccentricity/1
  Blob Extraction/7(blob_orientation) -> Orientation/1
  Blob Extraction/6(blob_minor_axis) -> MinorAxis/1
  Blob Extraction/5(blob_major_axis) -> MajorAxis/1
  Blob Extraction/4(blob_bbox) -> BBox/1
  Blob Extraction/3(blob_centroids) -> Centroid/1
  Blob Extraction/2(blob_area) -> Area/1
  Blob Extraction/1(blob_hues) -> BlobHues/1
  ColorFilter/1 -> Blob Extraction/4(ColorFilter)
  white_al/1 -> Blob Extraction/5(white_al)
  white_au/1 -> Blob Extraction/6(white_au)
  white_bl/1 -> Blob Extraction/7(white_bl)
  white_bu/1 -> Blob Extraction/8(white_bu)
  black_al/1 -> Blob Extraction/9(black_al)
  black_au/1 -> Blob Extraction/10(black_au)
  black_bl/1 -> Blob Extraction/11(black_bl)
  black_bu/1 -> Blob Extraction/12(black_bu)
  blue_au/1 -> Blob Extraction/14(blue_au)
  blue_bl/1 -> Blob Extraction/15(blue_bl)
  blue_bu/1 -> Blob Extraction/16(blue_bu)
  red_al/1 -> Blob Extraction/17(red_al)
  red_au/1 -> Blob Extraction/18(red_au)
  red_bl/1 -> Blob Extraction/19(red_bl)
  red_bu/1 -> Blob Extraction/20(red_bu)
  IterativeSegmentation/1(LabelMatrix) -> Blob Extraction/1(LabelMatrix), Segmented Image/1(LabelMatrix)
  IterativeSegmentation/2(num_colors) -> Blob Extraction/2(num_colors), num_colors/1
  IterativeSegmentation/3(ref_colors) -> Blob Extraction/3(ref_colors), Segmented Image/2(ref_colors), ref_colors/1
  Dist_Thresh/1 -> IterativeSegmentation/4(Iter_Segment_Thresh)
  R_in/1 -> IterativeSegmentation/1(R)
  G_in/1 -> IterativeSegmentation/2(G)
  B_in/1 -> IterativeSegmentation/3(B)
  If/1 -> Segmented Image/Action
  OutputSegmentedImage/1 -> If/1
  Segmented Image/1(R_out) -> R_out/1
  Segmented Image/2(G_out) -> G_out/1
  Segmented Image/3(B_out) -> B_out/1
  green_bu/1 -> Blob Extraction/32(green_bu)
  blue_al/1 -> Blob Extraction/13(blue_al)
  orange_al/1 -> Blob Extraction/21(orange_al)
  orane_au/1 -> Blob Extraction/22(orange_au)
  orange_bl/1 -> Blob Extraction/23(orange_bl)
  orange_bu/1 -> Blob Extraction/24(orange_bu)
  yellow_al/1 -> Blob Extraction/25(yellow_al)
  yellow_au/1 -> Blob Extraction/26(yellow_au)
  yellow_bl/1 -> Blob Extraction/27(yellow_bl)
  yellow_bu/1 -> Blob Extraction/28(yellow_bu)
  green_al/1 -> Blob Extraction/29(green_al)
  green_au/1 -> Blob Extraction/30(green_au)
  breen_bl/1 -> Blob Extraction/31(green_bl)

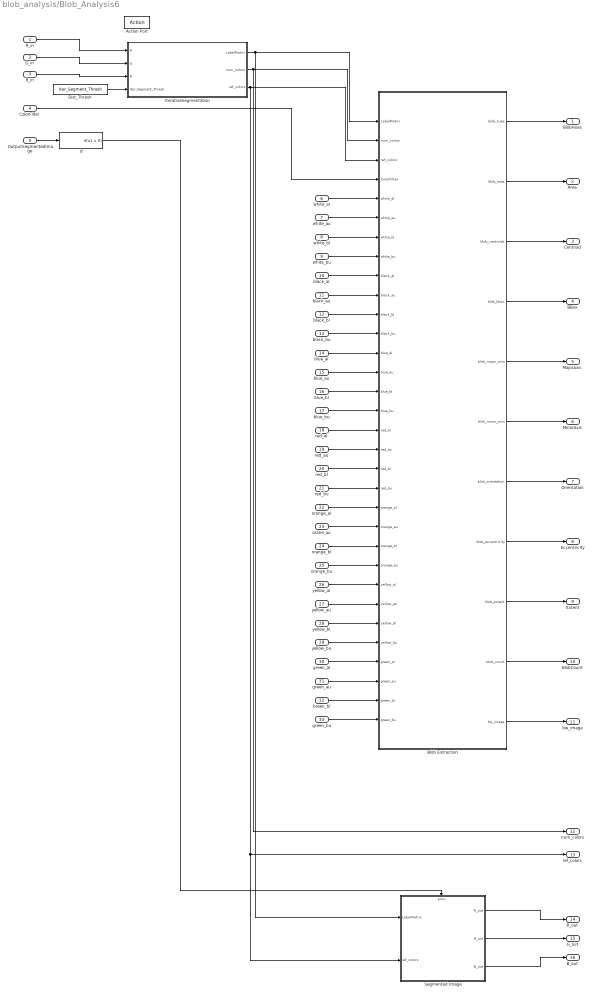
== system blob_analysis/Blob_Analysis6 ==
  R_in : Inport
  G_in : Inport  Port=2
  B_in : Inport  Port=3
  ColorFilter : Inport  Port=4
  OutputSegmentedImage : Inport  Port=5
  white_al : Inport  Port=6
  white_au : Inport  Port=7
  white_bl : Inport  Port=8
  white_bu : Inport  Port=9
  black_al : Inport  Port=10
  black_au : Inport  Port=11
  black_bl : Inport  Port=12
  black_bu : Inport  Port=13
  blue_al : Inport  Port=14
  blue_au : Inport  Port=15
  blue_bl : Inport  Port=16
  blue_bu : Inport  Port=17
  red_al : Inport  Port=18
  red_au : Inport  Port=19
  red_bl : Inport  Port=20
  red_bu : Inport  Port=21
  orange_al : Inport  Port=22
  orane_au : Inport  Port=23
  orange_bl : Inport  Port=24
  orange_bu : Inport  Port=25
  yellow_al : Inport  Port=26
  yellow_au : Inport  Port=27
  yellow_bl : Inport  Port=28
  yellow_bu : Inport  Port=29
  green_al : Inport  Port=30
  green_au : Inport  Port=31
  breen_bl : Inport  Port=32
  green_bu : Inport  Port=33
  Action Port : ActionPort
  Blob Extraction : Stateflow chart  TreatAsAtomicUnit=on
  Dist_Thresh : Constant  Value=Iter_Segment_Thresh  SampleTime=-1
  If : If  ShowElse=off
  IterativeSegmentation : Subsystem
      settings: UndoDeleteFcn=Stateflow.SLINSF.SimulinkMan.restorePreDeleteFcn  PreDeleteFcn=Stateflow.SLINSF.SimulinkMan.removePreDeleteFcn
  Segmented Image : Subsystem  TreatAsAtomicUnit=on
  BlobHues : Outport
  Area : Outport  Port=2
  Centroid : Outport  Port=3
  BBox : Outport  Port=4
  MajorAxis : Outport  Port=5
  MinorAxis : Outport  Port=6
  Orientation : Outport  Port=7
  Eccentricity : Outport  Port=8
  Extent : Outport  Port=9
  BlobCount : Outport  Port=10
  bw_image : Outport  Port=11
  num_colors : Outport  Port=12
  ref_colors : Outport  Port=13
  R_out : Outport  Port=14
  G_out : Outport  Port=15
  B_out : Outport  Port=16
  wires:
  Blob Extraction/11(bw_image) -> bw_image/1
  Blob Extraction/10(blob_count) -> BlobCount/1
  Blob Extraction/9(blob_extent) -> Extent/1
  Blob Extraction/8(blob_eccentricity) -> Eccentricity/1
  Blob Extraction/7(blob_orientation) -> Orientation/1
  Blob Extraction/6(blob_minor_axis) -> MinorAxis/1
  Blob Extraction/5(blob_major_axis) -> MajorAxis/1
  Blob Extraction/4(blob_bbox) -> BBox/1
  Blob Extraction/3(blob_centroids) -> Centroid/1
  Blob Extraction/2(blob_area) -> Area/1
  Blob Extraction/1(blob_hues) -> BlobHues/1
  ColorFilter/1 -> Blob Extraction/4(ColorFilter)
  white_al/1 -> Blob Extraction/5(white_al)
  white_au/1 -> Blob Extraction/6(white_au)
  white_bl/1 -> Blob Extraction/7(white_bl)
  white_bu/1 -> Blob Extraction/8(white_bu)
  black_al/1 -> Blob Extraction/9(black_al)
  black_au/1 -> Blob Extraction/10(black_au)
  black_bl/1 -> Blob Extraction/11(black_bl)
  black_bu/1 -> Blob Extraction/12(black_bu)
  blue_au/1 -> Blob Extraction/14(blue_au)
  blue_bl/1 -> Blob Extraction/15(blue_bl)
  blue_bu/1 -> Blob Extraction/16(blue_bu)
  red_al/1 -> Blob Extraction/17(red_al)
  red_au/1 -> Blob Extraction/18(red_au)
  red_bl/1 -> Blob Extraction/19(red_bl)
  red_bu/1 -> Blob Extraction/20(red_bu)
  IterativeSegmentation/1(LabelMatrix) -> Blob Extraction/1(LabelMatrix), Segmented Image/1(LabelMatrix)
  IterativeSegmentation/2(num_colors) -> Blob Extraction/2(num_colors), num_colors/1
  IterativeSegmentation/3(ref_colors) -> Blob Extraction/3(ref_colors), Segmented Image/2(ref_colors), ref_colors/1
  Dist_Thresh/1 -> IterativeSegmentation/4(Iter_Segment_Thresh)
  R_in/1 -> IterativeSegmentation/1(R)
  G_in/1 -> IterativeSegmentation/2(G)
  B_in/1 -> IterativeSegmentation/3(B)
  If/1 -> Segmented Image/Action
  OutputSegmentedImage/1 -> If/1
  Segmented Image/1(R_out) -> R_out/1
  Segmented Image/2(G_out) -> G_out/1
  Segmented Image/3(B_out) -> B_out/1
  green_bu/1 -> Blob Extraction/32(green_bu)
  blue_al/1 -> Blob Extraction/13(blue_al)
  orange_al/1 -> Blob Extraction/21(orange_al)
  orane_au/1 -> Blob Extraction/22(orange_au)
  orange_bl/1 -> Blob Extraction/23(orange_bl)
  orange_bu/1 -> Blob Extraction/24(orange_bu)
  yellow_al/1 -> Blob Extraction/25(yellow_al)
  yellow_au/1 -> Blob Extraction/26(yellow_au)
  yellow_bl/1 -> Blob Extraction/27(yellow_bl)
  yellow_bu/1 -> Blob Extraction/28(yellow_bu)
  green_al/1 -> Blob Extraction/29(green_al)
  green_au/1 -> Blob Extraction/30(green_au)
  breen_bl/1 -> Blob Extraction/31(green_bl)

== system blob_analysis/Blob Analysis/If Action Subsystem ==
  LabelMatrix : Inport
  num_colors : Inport  Port=2
  ref_colors : Inport  Port=3
  Action Port : ActionPort  ActionType=then
  Color Space  Conversion : vipconversions/Color Space  Conversion  conversion=Obsolete  conversionActive=L*a*b* to sR'G'B'  wp_str=D65  rec=Rec. 601 (SDTV)  sys=1125/60/2:1  imagePorts=Separate color signals
  Filter Image1 : Stateflow chart  TreatAsAtomicUnit=on
  R_out : Outport
  G_out : Outport  Port=2
  B_out : Outport  Port=3
  wires:
  LabelMatrix/1 -> Filter Image1/1(LabelMatrix)
  num_colors/1 -> Filter Image1/2(num_colors)
  ref_colors/1 -> Filter Image1/3(ref_colors)
  Filter Image1/1(L) -> Color Space  Conversion/1
  Filter Image1/2(a) -> Color Space  Conversion/2
  Filter Image1/3(b) -> Color Space  Conversion/3
  Color Space  Conversion/1 -> R_out/1
  Color Space  Conversion/2 -> G_out/1
  Color Space  Conversion/3 -> B_out/1

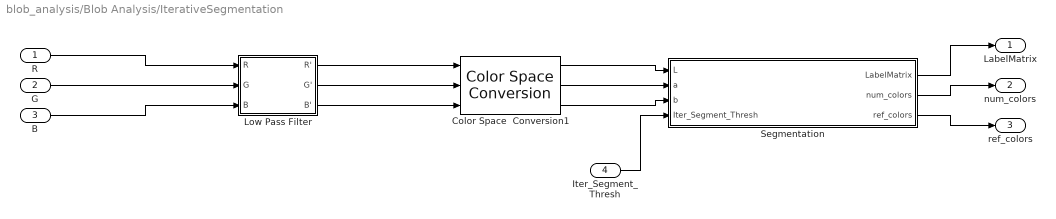
== system blob_analysis/Blob Analysis/IterativeSegmentation ==
  R : Inport
  G : Inport  Port=2
  B : Inport  Port=3
  Iter_Segment_Thresh : Inport  Port=4
  Color Space  Conversion1 : vipconversions/Color Space  Conversion  conversion=Obsolete  conversionActive=sR'G'B' to L*a*b*  wp_str=D50  rec=Rec. 601 (SDTV)  sys=1125/60/2:1  imagePorts=Separate color signals
  Low Pass Filter : Subsystem
  Segmentation : Subsystem
  LabelMatrix : Outport
  num_colors : Outport  Port=2
  ref_colors : Outport  Port=3
  wires:
  Low Pass Filter/3(B') -> Color Space  Conversion1/3
  Low Pass Filter/2(G') -> Color Space  Conversion1/2
  Low Pass Filter/1(R') -> Color Space  Conversion1/1
  Color Space  Conversion1/3 -> Segmentation/3(b)
  Color Space  Conversion1/2 -> Segmentation/2(a)
  Color Space  Conversion1/1 -> Segmentation/1(L)
  R/1 -> Low Pass Filter/1(R)
  G/1 -> Low Pass Filter/2(G)
  B/1 -> Low Pass Filter/3(B)
  Segmentation/1(LabelMatrix) -> LabelMatrix/1
  Segmentation/2(num_colors) -> num_colors/1
  Segmentation/3(ref_colors) -> ref_colors/1
  Iter_Segment_Thresh/1 -> Segmentation/4(Iter_Segment_Thresh)

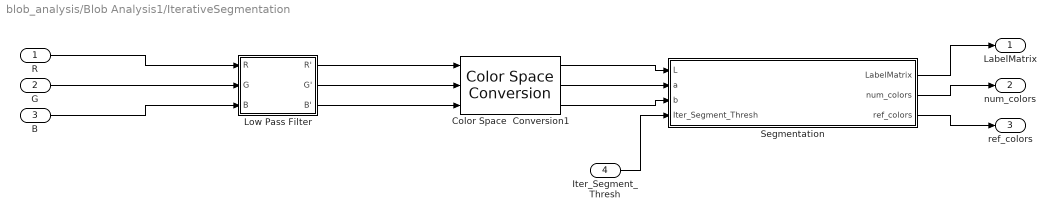
== system blob_analysis/Blob Analysis1/IterativeSegmentation ==
  R : Inport
  G : Inport  Port=2
  B : Inport  Port=3
  Iter_Segment_Thresh : Inport  Port=4
  Color Space  Conversion1 : vipconversions/Color Space  Conversion  conversion=Obsolete  conversionActive=sR'G'B' to L*a*b*  wp_str=D50  rec=Rec. 601 (SDTV)  sys=1125/60/2:1  imagePorts=Separate color signals
  Low Pass Filter : Subsystem
  Segmentation : Subsystem
  LabelMatrix : Outport
  num_colors : Outport  Port=2
  ref_colors : Outport  Port=3
  wires:
  Low Pass Filter/3(B') -> Color Space  Conversion1/3
  Low Pass Filter/2(G') -> Color Space  Conversion1/2
  Low Pass Filter/1(R') -> Color Space  Conversion1/1
  Color Space  Conversion1/3 -> Segmentation/3(b)
  Color Space  Conversion1/2 -> Segmentation/2(a)
  Color Space  Conversion1/1 -> Segmentation/1(L)
  R/1 -> Low Pass Filter/1(R)
  G/1 -> Low Pass Filter/2(G)
  B/1 -> Low Pass Filter/3(B)
  Segmentation/1(LabelMatrix) -> LabelMatrix/1
  Segmentation/2(num_colors) -> num_colors/1
  Segmentation/3(ref_colors) -> ref_colors/1
  Iter_Segment_Thresh/1 -> Segmentation/4(Iter_Segment_Thresh)

== system blob_analysis/Blob Analysis1/Segmented Image ==
  LabelMatrix : Inport
  ref_colors : Inport  Port=2
  Action Port : ActionPort  ActionType=then
  Color Space  Conversion : vipconversions/Color Space  Conversion  conversion=Obsolete  conversionActive=L*a*b* to sR'G'B'  wp_str=D65  rec=Rec. 601 (SDTV)  sys=1125/60/2:1  imagePorts=Separate color signals
  Display Image : Stateflow chart  TreatAsAtomicUnit=on
  R_out : Outport
  G_out : Outport  Port=2
  B_out : Outport  Port=3
  wires:
  LabelMatrix/1 -> Display Image/1(LabelMatrix)
  ref_colors/1 -> Display Image/2(ref_colors)
  Display Image/1(L) -> Color Space  Conversion/1
  Display Image/2(a) -> Color Space  Conversion/2
  Display Image/3(b) -> Color Space  Conversion/3
  Color Space  Conversion/1 -> R_out/1
  Color Space  Conversion/2 -> G_out/1
  Color Space  Conversion/3 -> B_out/1

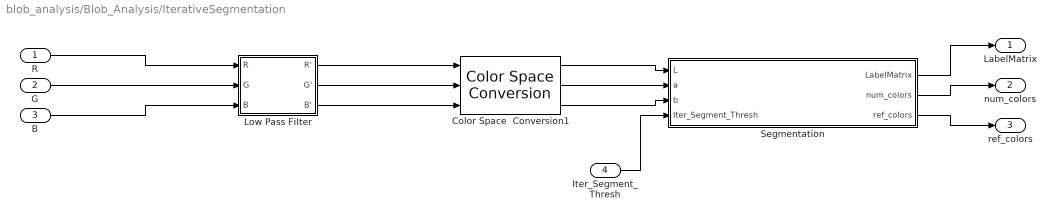
== system blob_analysis/Blob_Analysis/IterativeSegmentation ==
  R : Inport
  G : Inport  Port=2
  B : Inport  Port=3
  Iter_Segment_Thresh : Inport  Port=4
  Color Space  Conversion1 : vipconversions/Color Space  Conversion  conversion=Obsolete  conversionActive=sR'G'B' to L*a*b*  wp_str=D50  rec=Rec. 601 (SDTV)  sys=1125/60/2:1  imagePorts=Separate color signals
  Low Pass Filter : Subsystem
  Segmentation : Subsystem
  LabelMatrix : Outport
  num_colors : Outport  Port=2
  ref_colors : Outport  Port=3
  wires:
  Iter_Segment_Thresh/1 -> Segmentation/4(Iter_Segment_Thresh)
  Segmentation/3(ref_colors) -> ref_colors/1
  Segmentation/2(num_colors) -> num_colors/1
  Segmentation/1(LabelMatrix) -> LabelMatrix/1
  B/1 -> Low Pass Filter/3(B)
  G/1 -> Low Pass Filter/2(G)
  R/1 -> Low Pass Filter/1(R)
  Color Space  Conversion1/1 -> Segmentation/1(L)
  Color Space  Conversion1/2 -> Segmentation/2(a)
  Color Space  Conversion1/3 -> Segmentation/3(b)
  Low Pass Filter/1(R') -> Color Space  Conversion1/1
  Low Pass Filter/2(G') -> Color Space  Conversion1/2
  Low Pass Filter/3(B') -> Color Space  Conversion1/3

== system blob_analysis/Blob_Analysis/Segmented Image ==
  LabelMatrix : Inport
  ref_colors : Inport  Port=2
  Action Port : ActionPort  ActionType=then
  Color Space  Conversion : vipconversions/Color Space  Conversion  conversion=Obsolete  conversionActive=L*a*b* to sR'G'B'  wp_str=D65  rec=Rec. 601 (SDTV)  sys=1125/60/2:1  imagePorts=Separate color signals
  Display Image : Stateflow chart  TreatAsAtomicUnit=on
  R_out : Outport
  G_out : Outport  Port=2
  B_out : Outport  Port=3
  wires:
  Color Space  Conversion/3 -> B_out/1
  Color Space  Conversion/2 -> G_out/1
  Color Space  Conversion/1 -> R_out/1
  Display Image/3(b) -> Color Space  Conversion/3
  Display Image/2(a) -> Color Space  Conversion/2
  Display Image/1(L) -> Color Space  Conversion/1
  ref_colors/1 -> Display Image/3(ref_colors)
  LabelMatrix/1 -> Display Image/1(LabelMatrix)

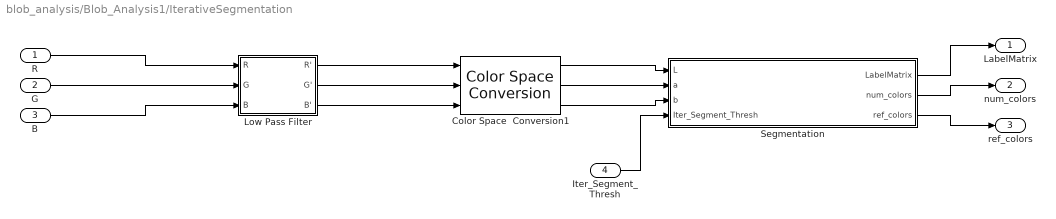
== system blob_analysis/Blob_Analysis1/IterativeSegmentation ==
  R : Inport
  G : Inport  Port=2
  B : Inport  Port=3
  Iter_Segment_Thresh : Inport  Port=4
  Color Space  Conversion1 : vipconversions/Color Space  Conversion  conversion=Obsolete  conversionActive=sR'G'B' to L*a*b*  wp_str=D50  rec=Rec. 601 (SDTV)  sys=1125/60/2:1  imagePorts=Separate color signals
  Low Pass Filter : Subsystem
  Segmentation : Subsystem
  LabelMatrix : Outport
  num_colors : Outport  Port=2
  ref_colors : Outport  Port=3
  wires:
  Low Pass Filter/3(B') -> Color Space  Conversion1/3
  Low Pass Filter/2(G') -> Color Space  Conversion1/2
  Low Pass Filter/1(R') -> Color Space  Conversion1/1
  Color Space  Conversion1/3 -> Segmentation/3(b)
  Color Space  Conversion1/2 -> Segmentation/2(a)
  Color Space  Conversion1/1 -> Segmentation/1(L)
  R/1 -> Low Pass Filter/1(R)
  G/1 -> Low Pass Filter/2(G)
  B/1 -> Low Pass Filter/3(B)
  Segmentation/1(LabelMatrix) -> LabelMatrix/1
  Segmentation/2(num_colors) -> num_colors/1
  Segmentation/3(ref_colors) -> ref_colors/1
  Iter_Segment_Thresh/1 -> Segmentation/4(Iter_Segment_Thresh)

== system blob_analysis/Blob_Analysis1/Segmented Image ==
  LabelMatrix : Inport
  ref_colors : Inport  Port=2
  Action Port : ActionPort
  Color Space  Conversion : vipconversions/Color Space  Conversion  conversion=Obsolete  conversionActive=L*a*b* to sR'G'B'  wp_str=D65  rec=Rec. 601 (SDTV)  sys=1125/60/2:1  imagePorts=Separate color signals
  Display Image : Stateflow chart  TreatAsAtomicUnit=on
  R_out : Outport
  G_out : Outport  Port=2
  B_out : Outport  Port=3
  wires:
  LabelMatrix/1 -> Display Image/1(LabelMatrix)
  ref_colors/1 -> Display Image/2(ref_colors)
  Display Image/1(L) -> Color Space  Conversion/1
  Display Image/2(a) -> Color Space  Conversion/2
  Display Image/3(b) -> Color Space  Conversion/3
  Color Space  Conversion/1 -> R_out/1
  Color Space  Conversion/2 -> G_out/1
  Color Space  Conversion/3 -> B_out/1

== system blob_analysis/Blob_Analysis2/IterativeSegmentation ==
  R : Inport
  G : Inport  Port=2
  B : Inport  Port=3
  Iter_Segment_Thresh : Inport  Port=4
  Color Space  Conversion1 : vipconversions/Color Space  Conversion  conversion=Obsolete  conversionActive=sR'G'B' to L*a*b*  wp_str=D50  rec=Rec. 601 (SDTV)  sys=1125/60/2:1  imagePorts=Separate color signals
  Low Pass Filter : Subsystem
  Segmentation : Subsystem
  LabelMatrix : Outport
  num_colors : Outport  Port=2
  ref_colors : Outport  Port=3
  wires:
  Low Pass Filter/3(B') -> Color Space  Conversion1/3
  Low Pass Filter/2(G') -> Color Space  Conversion1/2
  Low Pass Filter/1(R') -> Color Space  Conversion1/1
  Color Space  Conversion1/3 -> Segmentation/3(b)
  Color Space  Conversion1/2 -> Segmentation/2(a)
  Color Space  Conversion1/1 -> Segmentation/1(L)
  R/1 -> Low Pass Filter/1(R)
  G/1 -> Low Pass Filter/2(G)
  B/1 -> Low Pass Filter/3(B)
  Segmentation/1(LabelMatrix) -> LabelMatrix/1
  Segmentation/2(num_colors) -> num_colors/1
  Segmentation/3(ref_colors) -> ref_colors/1
  Iter_Segment_Thresh/1 -> Segmentation/4(Iter_Segment_Thresh)

== system blob_analysis/Blob_Analysis2/Segmented Image ==
  LabelMatrix : Inport
  ref_colors : Inport  Port=2
  Action Port : ActionPort
  Color Space  Conversion : vipconversions/Color Space  Conversion  conversion=Obsolete  conversionActive=L*a*b* to sR'G'B'  wp_str=D65  rec=Rec. 601 (SDTV)  sys=1125/60/2:1  imagePorts=Separate color signals
  Display Image : Stateflow chart  TreatAsAtomicUnit=on
  R_out : Outport
  G_out : Outport  Port=2
  B_out : Outport  Port=3
  wires:
  LabelMatrix/1 -> Display Image/1(LabelMatrix)
  ref_colors/1 -> Display Image/2(ref_colors)
  Display Image/1(L) -> Color Space  Conversion/1
  Display Image/2(a) -> Color Space  Conversion/2
  Display Image/3(b) -> Color Space  Conversion/3
  Color Space  Conversion/1 -> R_out/1
  Color Space  Conversion/2 -> G_out/1
  Color Space  Conversion/3 -> B_out/1
